simulink model "matlabfunc"  (R2018a)
settings: Solver=FixedStepAuto  StartTime=0.0  StopTime=1e-3  FixedStep=1e-6  RelTol=1e-3
settings Model: Creator=user  LastModifiedBy=user

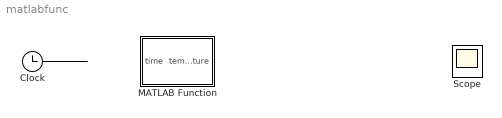
== system matlabfunc ==
  Clock : Clock
  MATLAB Function : MATLAB Function  TreatAsAtomicUnit=on
  Scope : Scope
  wires:
  Clock/1 -> ?
  ? -> Scope/1

== matlab function matlabfunc/MATLAB Function ==
  data: time input; temperature output
function temperature = calculateTemp(time)
L=5;
rho=2.70;
k=0.497;
c=0.215;

alpha=k/(rho*c);
scale=1e5;
if(time>0)
    temperature=erfc( L./(2*sqrt(alpha*time*scale)));
else
    temperature = time;
end
end
